simulink model "lab3"  (R2024a)
settings: Solver=VariableStepAuto  StartTime=0.0  StopTime=10  RelTol=1e-3
undefined symbols (not defined in the file): reg_num, T, T_1, T_2
settings Model: Creator=vladislav  LastModifiedBy=vladislav

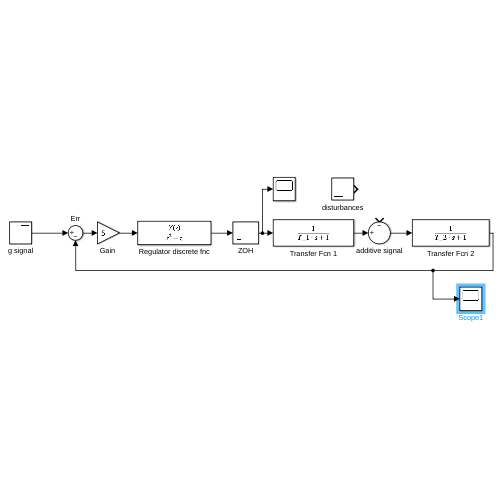
[thumbnail: Simulink's stored preview of the top-level diagram]
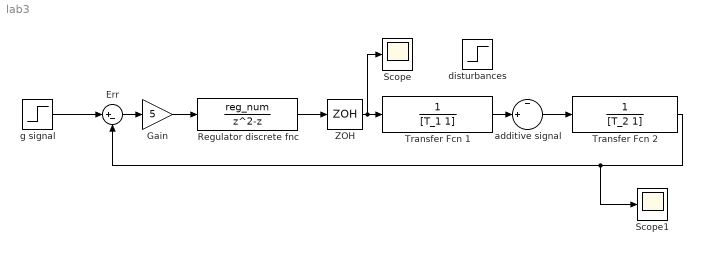
== system lab3 ==
  Err : Sum  Inputs=|+-
  "Gain " : Gain  Gain=5
  Regulator discrete fnc : DiscreteTransferFcn  Numerator=reg_num  Denominator=[1 -1 0]
  Scope : Scope
  Scope1 : Scope
  Transfer Fcn 1 : TransferFcn  Denominator=[T_1 1]
  Transfer Fcn 2 : TransferFcn  Denominator=[T_2 1]
  ZOH : ZeroOrderHold  SampleTime=T
  additive signal : Sum  Inputs=-|+||
  disturbances : Step  Before=1  SampleTime=0
  g signal : Step  Before=1  SampleTime=0
  wires:
  Err/1 -> "Gain "/1
  "Gain "/1 -> Regulator discrete fnc/1
  Regulator discrete fnc/1 -> ZOH/1
  ZOH/1 -> Scope/1, Transfer Fcn 1/1
  additive signal/1 -> Transfer Fcn 2/1
  Transfer Fcn 2/1 -> Scope1/1, Err/2
  Transfer Fcn 1/1 -> additive signal/2
  g signal/1 -> Err/1
